simulink model "sfcndemo_sfun_quantize"  (Simulink 7.6)
settings: Solver=FixedStepDiscrete  StartTime=0.0  StopTime=10.0  FixedStep=0.01  RelTol=1e-3
Description:
  | Vectorized Quantizer C-MEX S-function
settings Model: Creator=The MathWorks Inc.  ExtModeTrigMode=oneshot  ExtModeArmWhenConnect=off  ExtModeAutoUpdateStatusClock=off
settings DataIOCC: LimitDataPoints=off
settings OptimizationCC: BlockReduction=off  BooleanDataType=off  InitFltsAndDblsToZero=on
settings DebuggingCC: SaveWithParameterizedLinksMsg=none  SignalResolutionControl=TryResolveAllWithWarning  SolverPrmCheckMsg=none  MultiTaskDSMMsg=warning  MultiTaskCondExecSysMsg=none
settings HardwareCC: TargetUnknown=on
settings RTWCC: IncludeERTFirstTime=on
settings CodeAppCC: CustomSymbolStrFcn=$F$N$M
settings GRTTargetCC: TargetFcnLib=ansi_tfl_tmw.mat

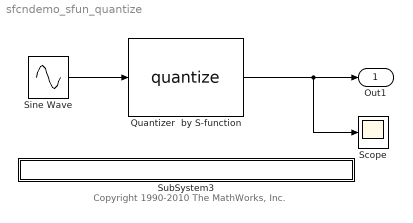
== system sfcndemo_sfun_quantize ==
  note: Copyright 1990-2010 The MathWorks, Inc.
  Quantizer  by S-function : S-Function  FunctionName=quantize  Parameters=q  EnableBusSupport=off  mask(S-function: sfun_quantize){q=2}
      mask prompts: q "Quantization interval:"
      mask help: This is a vectorized quantizer block. It quantizes the input into steps as specified by the quantization interval parameter, q.
      mask Display: plot([-.3 NaN 0 .4 0.8 1.2 1.6 2 2.4 2.8 3.2 3.6 4 4.4 4.8 5.2 5.6 6 6.4 6.8 7.2 7.6 8 8.4 8.8 9.2 9.6 10 NaN 10.3 NaN -.3 10.3 NaN 4 4],[-2.5 NaN 0 0 1 1 2 2 1 1 0 0 -1 -1 -2 -2 -1 -1 0 0 1 1 2 2 1 1 0 0 NaN 2.5 NaN 0 0 NaN -2.5 2.5]);
  Scope : Scope
      settings: TimeRange=10  YMin=-2  YMax=2
  Sine Wave : Sin  Amplitude=[1 2]  SampleTime=0
  SubSystem3 : Subsystem  mask{filename=quantize.c}
      mask init:
      | x=sfundemo_maskdisp;
      settings: AttributesFormatString=\n  OpenFcn=sfundemo_openfcn
      mask Display: disp(x);
  Out1 : Outport  InitialOutput=0
  wires:
  Sine Wave/1 -> Quantizer  by S-function/1
  Quantizer  by S-function/1 -> Out1/1, Scope/1

== system sfcndemo_sfun_quantize/SubSystem3 ==
